simulink model "GuytonModel1986All_R2015a"  (R2015a)
settings: Solver=ode15s  StartTime=0  StopTime=383040  FixedStep=0.03  MaxStep=360  RelTol=1e-3
libraries: simulink x3
(part 1 of 5)
settings Model: Creator=Jirka  LastModifiedBy=User
settings SolverCC: ZeroCrossControl=DisableAll  SolverResetMethod=Robust
settings DataIOCC: SignalLoggingSaveFormat=ModelDataLogs
settings OptimizationCC: ExpressionDepthLimit=2147483647  InitFltsAndDblsToZero=on
settings DebuggingCC: AlgebraicLoopMsg=error  ArtificialAlgebraicLoopMsg=error  SaveWithParameterizedLinksMsg=none  UnderspecifiedInitializationDetection=Classic  MergeDetectMultiDrivingBlocksExec=none  SignalResolutionControl=TryResolveAllWithWarning  SolverPrmCheckMsg=warning  MultiTaskDSMMsg=warning  MultiTaskCondExecSysMsg=none  FcnCallInpInsideContextMsg=EnableAllAsWarning  StateNameClashWarn=warning
settings GRTTargetCC: TargetFcnLib=ansi_tfl_tmw.mat  GeneratePreprocessorConditionals=Use local settings  CombineOutputUpdateFcns=off  GRTInterface=on

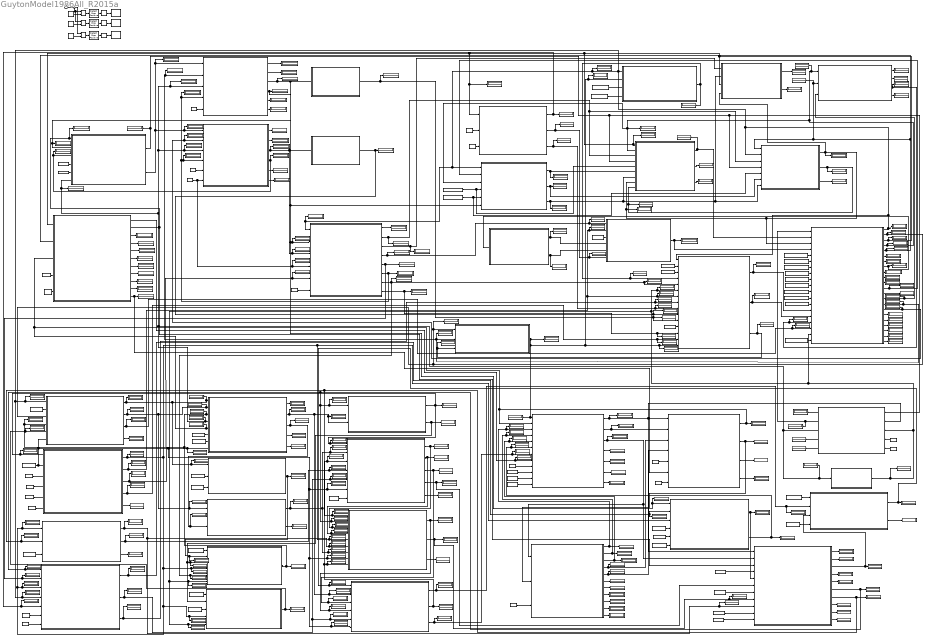
== system GuytonModel1986All_R2015a ==
  note: HSR
  note: HPR
  note: HPL
  2 : Constant
  AARK : Constant  Value=40
  ADH : Constant  Value=0
  AHMRM : Constant  Value=0
  ALCLK : Constant
  ALD : Constant  Value=0
  ANG : Constant  Value=0
  ANUBRM : Constant  Value=0
  ANUVM1 : Constant  Value=0
  ANXM : Constant  Value=0
  ANY : Constant  Value=-0.2
  ATRRFBM : Constant  Value=0
  ATRVFBM : Constant  Value=0
  AUZ : Constant
  Afferent Arteriole : Subsystem
      settings: MinAlgLoopOccurrences=on
      mask Display: disp('AFFERENT ARTERIOLE\n\nINTPUTS:\nAARK - normal resistance in afferent arteriole [torr min/l]\nRNAUG1 - macula densa feedback signal [ratio to normal] \nAUM - sympathetic vasoconstrictor effect on arteries \n[ratio to normal] \nANM - angiotensin multiplier effect on vascular resistance \n[ratio to normal]\nVIM - blood viscosity [ratio to normal blood] \n\n\n OUTPUT:\nAAR - afferent arteriolar resistance [torr l/min]\n')
  Assertion : Assertion  AssertionFailFcn=set_param(bdroot,'SimulationCommand','pause');  StopWhenAssertionFail=off
  Assertion1 : Assertion  AssertionFailFcn=set_param(bdroot,'SimulationCommand','pause');  StopWhenAssertionFail=off
  Assertion2 : Assertion  AssertionFailFcn=set_param(bdroot,'SimulationCommand','pause');  StopWhenAssertionFail=off
  Autonomic Contorl of the Circulation : Subsystem
      mask Display: disp('AUTONOMIC CONTROL OF THE CIRCULATION\n\nINTPUTS:\nPA - systemic arterial pressure torr\nPOT - non-muscle cell PO2 [torr]\nPMO - muscle cells PO2 [torr] \nEXC - Effect of excercise on the metabolic usage of oxygen \nby the muscles [ratio to resting state]\nANUBR - direct effect of angiotensin on vasomotor center \n["virtual" torr]\nAUZ - overall sensitivity of autonomic control [ratio to normal]\n\nOUTPUTs:\nAU - overall activity af autonomic system\n[ratio to normal]\nAUH - autonomic multilier effect on the heart output\n[ratio to normal]\nAUR - autonomic multilier effect on heart rate\n[ratio to normal]\nVVR - basic volume of venous tree(maximum volume\n at zero pressure) [l]\nAUP - autonomic multipllier effect on ADH hormone excretion etc. \n[ratio to normal]\nAOM - autonomic multipllier effect on tissue oxygen utilisation \n[ratio to normal]\nAUM - autonomic multipllier effect on arterial resistance \n[ratio to normal]\nAVE - autonomic multipllier effect on venous resistance\n[ratio to normal]\n')
  Blood viscosity : Subsystem
      settings: MinAlgLoopOccurrences=on
      mask Display: disp('BLOOD VISCOSITY\n\nINTPUT:\nHM - hematocrit [%]\n\nOUTPUT:\nVIM - blood viscosity [ratio to normal]')
  CAS : Constant  Value=0.00355
  "CFC " : Constant  Value=0.01167
  CLA : Constant  Value=0.01
  CPA : Constant  Value=0.0048
  CPF : Constant  Value=0.0003
  CPP : Constant  Value=72
  CRA : Constant  Value=0.005
  CV : Constant  Value=0.0825
  Capillary Membrane Fluid Dynamics : Subsystem
      mask Display: disp('CAPILLARY MEMBRANE FLUID DYNAMICS\n\nINTPUTS:\nPC - systemic capillary pressure [torr]\nPGH - hydrostatic pressure in the tissue gel [torr]\nPPC - plasma colloid osmotic pressure [torr] \nPTC - colloid osmotic pressure of the tissue gel [torr]\nVTL - rate of return of fluid from the interstitium to the\nblood through the lymph [l/min]\nTVD - rate of intake of fluid by mounth or otherwise [l/min]\nVUD - loss of fluid into the urine [l/min]\nDFP - loss of fluid from the pulmonary capillaries [l/min]\nVID - rate of transfer of fluid into the cells [l/min]\nCFC - capillary filtration coefficient [l/min/torr]\n(normal value CFC=0.01167)\nVPN - normal value of plasma volume [l]\nVTSN - normal value of interstitital fluid volume [l]/n\nOUTPUTS:\nVP - plasma volume [l]\nVTS - total interstitial fluid volume [l]\nVTCPL - rate of leakage of whole plasma through \n the capillary membrane [l/min]\nCFILTR - rate of filtration from the systemic capillaries [l/min]\nVTC - toral rate of movement of fluid out of systemic capillaries[l/min]\nVPR - plasma volume [ratio to normal]\nVTS - total interstitial fluid volume [ratio to normal]\n')
  Circulatory Dynamics - Flows And Pressures : Subsystem
      settings: MinAlgLoopOccurrences=on
      mask Display: disp('CIRCULATORY DYNAMICS - FLOWS AND PRESSURES\n\nINPUTS:\nVB - blood volume [l]\nQRO - actual right ventricular output [l/min]\nQLO - output of left ventricle [l/min]\nVVS0 - unstressed venous systemic vascular volume [l]\nVAS0 - unstressed volume in systemic arteries [l]\nVRA0 - unstressed right atrial volume [l]\nVPA0 - unstressed volume in pulmonary arteries [l]\nVLA0 - unstressed volume in left atrium and pulmonary veins [l] \nCAS - capacitance of systemic arteries [l/torr] \nCV - capacitance of venous systemic volume [l/torr] \nCRA - capacitance of right atrium [l/torr]\n CPA - capacitance of pulmonary arteries [l/torr]\n CLA - capacitance of left atrium and pulmonary veins [l/torr] \nRSN - vascular resistance in non-muscle \n and non renal tissues [torr min /l]\nRSM - vascular resistance in muscles [torr min /l]\n RPT -pulmonary vascular resistance [torr min /l] \nRR - total renal resistance [torr min /l]\nVIM - blood viscosity (ratio to normal blood)\nFIS - conductance of the fistula [l/min/torr]\n\nOUTPUTS: \nPA - arterial (aortic) pressure [torr]\nPVS - average venous pressure [torr]\nPRA - right atrial pressure [torr]\nPPA - pulmonary arterial pressure [torr]\nPLA - left atrial pressure [torr]\nVAS - volume in systemic arteries [l]\nVVS - systemic venous vascular volume [l]\nVVE - excess blood volume in the veins [l] \nVRA - right atrial volume [l]\nVPA - volume in pulmonary arteries [l]\nVLA - volume in left atrium [l]\nQAO - blood flow in the systemic arterial system [l/min]\nQVO - rate of blood flow from veins into right atrium [l/min]\nQPO - rate of blood flow into pulmonary veins\n and left atrium [l/min]\nBFN - blood flow in non muscle and non renal tissues [l/min]\nBFM - blood flow in muscles [l/min]\nRBF - renal blood flow [l/min]\nFISFLO - blood flow through a fistula [l/min]\nRTP - total systemic peripheral resistance [torr min /l]\nVT0 - total unstressed blood volume [l]	\nVE0 - total excess volume of blood in the vasculature [l]\nMCP - mean circulatory pressure [torr]\n');
  Clock : Clock
  Constant : Constant  Value=20160
  Constant1 : Constant  Value=40320
  Constant137 : Constant  Value=30240
  DIURET : Constant
  DPR : Constant  Value=0
  DR : Constant  Value=0
  "Delivery of Oxygen to the Muscles " : Subsystem
      settings: MinAlgLoopOccurrences=on
      mask Display: disp('MUSCLE O2 DELIVERY\n\nINTPUTS:\nOVA - oxygen content of arterial blood \n[ml O2 STPD/l blood] \nBFN - blood flow in muscles \n [l/min]\nHM - hematocrit [%]\n    AOM - autonomic effect on tissue oxygenation \n [ratio to normal]\nOMM - basic oxygen utilisation in muscles \n[ml O2 STPD/min]\nEXC - Effect of excercise on the metabolic usage \nof oxygen by the muscles [ratio to resting state]\n\nOUTPUTS:\nOVS - muscle venous oxygen saturation [%]\nPVO - muscle venous PO2 [torr]\nPMO - muscle cell PO2 [torr]\nRMO - rate of oxygen delivery to muscles \n[ml O2 STPD/min]\nMMO - rate of oxygen utilisation by muscles\n[ml O2 STPD/min]\nQOM - muscle total cellular oxygen \n[ml O2 STPPD]\n')
  Delivery of Oxygen to the Non-muscleTtissues : Subsystem
      settings: MinAlgLoopOccurrences=on
      mask Display: disp('NON MUSCLE O2 DELIVERY\n\nINTPUTS:\nOVA - oxygen content of arterial blood \n[ml O2 STPD/l blood] \nBFN - blood flow in non-muscle and non-renal tissues \n [l/min]\nHM - hematocrit [%]\n    AOM - autonomic effect on tissue oxygenation \n[ratio to normal]\nO2M - basic oxygen utilisation in non-muscle cells \n[ml O2 STPD/min]\n\nOUTPUTS:\nOSV - non-muscle venous oxygen saturation [%]\nPOV - non muscle venous PO2 [torr]\nPOT - non muscle cell PO2 [torr]\nDOB - rate of oxygen delivery to non-muscle cells \n[ml O2 STPD/min]\nMO2 - rate of oxygen utilisation by non-muscle tissues \n[ml O2 STPD/min]\nQO2 - non-muscle total cellular oxygen \n[ml O2 STPD]\n')
  Detect Rise Positive : simulink/Logic and Bit Operations/Detect Rise Positive  vinit=0  InputProcessing=Inherited  OutDataTypeStr=boolean
  Detect Rise Positive1 : simulink/Logic and Bit Operations/Detect Rise Positive  vinit=0  InputProcessing=Inherited  OutDataTypeStr=boolean
  Detect Rise Positive2 : simulink/Logic and Bit Operations/Detect Rise Positive  vinit=0  InputProcessing=Inherited  OutDataTypeStr=boolean
  Display{,1..266} (267 alike) : Display
  EARK : Constant  Value=43.333
  EFARF : Constant  Value=0
  EXC : Constant
  Effect of stress relaxation on basic venous volume : Subsystem
      settings: MinAlgLoopOccurrences=on
      mask Display: disp('VENOUS STRESS RELAXATION\n\nINTPUTS:\nVVE - excess blood volume in the veins [l] \n\nOUTPUTS:\nVV6 - increased venous vascular volume \ncaused by long time stress realaxation [l]\nVV7 - - increased venous vascular volume \ncaused by short time stress realaxation [l]\n')
  Efferent Arteriole : Subsystem
      settings: MinAlgLoopOccurrences=on
      mask Display: disp('EFFERENT ARTERIOLE\n\nINTPUTS:\nAARK - normal resistance in efferent arteriole [torr min/l\nRNAUG1 - macula densa feedback signal \nto efferent arteriole [ratio to normal] \nEAFRF - sensitivity contoller of macula densa feedback signal\nto efferent arteriole\nANM - angiotensin multiplier effect on vascular resistance \n[ratio to normal]\nVIM - blood viscosity [ratio to normal blood] \n\n\n OUTPUT:\nAAR - afferent arteriolar resistance [torr l/min]\n')
  Extracellular and Intracellular Fluid Electrolytes and Volumes : Subsystem
      settings: MinAlgLoopOccurrences=on
      mask Display: disp('ECF AND ICF ELECTROLYTES AND VOLUMES\n\nINTPUTS:\nVP - plasma volume [l]\nVTS - systemic interstitial fluid volume [l]\nVPF - pulmonary interstitial fluid volume [l]\nNID - normal rate of sodium intake [mmol/min]\nSTH - salt appetite multiplier factor [ratio to normal]\nNOD - rate of excretion of sodium in the urine [mmol/min]\nKID - rate of intake of potassium [mmol/min]\nKOD - rate of excretion of potassium in the urine [mmol/min]\nAMK - aldosterone multiplier factor for the effect of aldosterone \n on the transport of potassium\n through the cell membrane [ratio of normal effect]\nACLK - sensitivity control of the effect of the aldosterone \n on cellular membrane transport\n of potassium [ratio of normal effect]\nVICnorm - normal value of the intracellular fluid volume [l]\n \nOUTPUTS:\nVEC - volume of extracellular fluid [l]\nVIC - volume of intracellular fluid [l]\nVTW - total body water [l]\nVID - rate of fluid transfer between interstitial fluid and cells [l/min]\nNAE - total extracellular sodium content [mmol]\nCNA - extracellular sodium concentration [mmol/l]\nCKE - extracellular potassium concentration [mmol/l]\nKI - total intracellular potassium content [mmol]\nCKI - intracellular potassium concentration [mmol/l]\nKCD - rate of transferof potassium from the interstitial fluid \ninto the intracellular fluid [mmol/min]\n')
  FIS : Constant  Value=0
  GBL : Constant  Value=0
  GLFC : Constant  Value=0.0208
  Glomerulus : Subsystem
      settings: MinAlgLoopOccurrences=on
      mask Display: disp('GLOMERULUS\n\nINTPUTS:\nPAR - renal perfusion pressure[torr]\nRFN - renal blood flow if kidney is not damaged [l/min] \nAAR - resistance in afferent arteriole \n[torr min/ll] \nHM - hematocrit \nPPC - plasma colloid osmotic pressure [torr]\nPXTP - back pressurein proximal tubule [torr]\nGLFC - glomerular filtration coefficient [l/torr/min]\nREK - percent of normal renal function [ratio to normal] \n\n\n OUTPUTS:\nGFR - glomerular filtration rate [l/min]\nGFN - glomerular filtration rate if kidney is not damaged [l/min]\nGLP - glomerular pressure [torr]\nGLPC - average glomerular plasma colloid osmotic pressure [torr]\nPFL - net pressure gradient in glomerulus [torr]\n')
  HSL : Constant
  HSR : Constant
  Heart Rate and Stroke Volume : Subsystem
      settings: MinAlgLoopOccurrences=on
      mask Display: disp('HEART RATE AND STROKE VOLUME\n\nINTPUTS:\nAUR - autonomic stimulation of heart rate \n[ratio to normal] \nHMD - cardiac depresant effect of hypoxia, shock\nand other factors [ratio to normal] \nPRA - right atrial pressure [torr]\nQLO - output of left ventricle [l/min]\n\nOUTPUTS:\nHR - heart rate [beats/min]\nSVO - stroke volume [l]\n')
  Heart hypertrophy or deterioration : Subsystem
      settings: MinAlgLoopOccurrences=on
      mask Display: disp('HEART HYPERTROPHY OR DETERIORATION\n\nINTPUTS:\nPA - systemic arterial pressure [torr]\nQAO - blood flow in the systemic arteriel system [l/min]\nPPA - pulmonary arterial pressure [torr]\nHSR - basic strenght or right ventricle [ratio to normal]\nHSL - basic strenght or left ventricle [ratio to normal]\nPOT - Non muscle cells PO2 [troo]\n\nOUTPUTS:\nHPR - hypertrophy effect of right heart [ratio to normal]\nHPL - hypertrophy effect of left heart [ratio to normal]\nHMD - cardiac depresant effect of hypoxia, shock\n')
  "Interstitial Tissue Fluids, Pressures and Gel Dynamics" : Subsystem
      mask Display: disp('INTERSTITIAL TISSUE FLUIDS, PRESSURES AND PROTEIN DYNAMICS\n\nINTPUTS:\nVTS - total interstitial fluid volume [l]\nDPC -rate of influx protein into the interstitial fluid from plasma [g/min]\nTSP0 - initial value of total interstitial tissue proteins [g]\n\nOUTPUTs:\nPGH - hydrostatic pressure in tissue gel [torr]\nPTC - total colloid osmotic pressure of the tissue gel]\nVTL - lymph flow rate [l/min]\nDPL - rate of return of protein to the circulatin by way of the lymph [g/min]\nCPI - concentration pf protein in the interstitium [g/l]\nPTT - total interstitial tissue pressure [torr]\nPIF - pressurte in the free interstitial fluid [torr]\nPTS - solid tissue pressure [torr]\nVIF - free interstitial fluid volume[l]\nVG - tissue gel volume[l]\nTSP - total interstitial tissue proteins [g]\n')
  KID : Constant  Value=0.06
  LPPR : Constant  Value=0.03
  Left Heart Pumping : Subsystem
      settings: MinAlgLoopOccurrences=on
      mask Display: disp('LEFT HEART PUMPING\n\nINTPUTS:\nPLA - left atrial pressure [torr]\nPA - systemic arterial pressure [torr]\nAUH - autonomic stimulation of heart [ratio to normal] \nOSA - oxygen hemoglobin saturation \nHSL - basic strenght or left ventricle (ratio to normal)\nHPL - hypertrophy effect of left heart [ratio to normal]\nHMD - cardiac depressant effect of hypoxia, shock \n and other factors [ratio to normal]\n\nOUTPUTS:\nQLO - actual left ventricular output [l/min]\nQLN - normalised lwft ventricular output [l/min]\nLVM - depressing effect on left ventricle of pulmonary \n arterial pressure [ratio to normal]\n')
  Logical Operator : Logic  Operator=NOT  AllPortsSameDT=off  OutDataTypeStr=boolean
  Logical Operator1 : Logic  Operator=NOT  AllPortsSameDT=off  OutDataTypeStr=boolean
  Logical Operator2 : Logic  Operator=NOT  AllPortsSameDT=off  OutDataTypeStr=boolean
  MYOGTAU : Constant  Value=240
  MYOGTAU1 : Constant  Value=240
  Macula densa : Subsystem
      settings: MinAlgLoopOccurrences=on
      mask Display: disp('MACULA DENSA\n\nINTPUTS:\nCNA - Extracellular sodium concentration [mmol/l]\nGFN - glomerular filtration rate if kidney \nis not damaged [l/min]\n\n\n OUTPUTS:\nRNAUG1 - macula densa feedback signal \n[ratio to normal effect]\nNAPT1 - delivery of sodium to the macula densa area \n[ratio to normal value]\n')
  "Muscle Local Blood Flow Control " : Subsystem
      settings: MinAlgLoopOccurrences=on
      mask Display: disp('MUSCLE LOCAL BLOOD FLOW CONTROL\n\nINTPUT:\nPMO - muscle cells PO2 [torr] \n\nOUTPUT:\nAMM - vasoconstrictor effect of local blood flow\n autoregulationin muscles\n[ratio to normal]\n')
  Myogenic Autoregulation : Subsystem
      settings: MinAlgLoopOccurrences=on
      mask Display: disp('MYOGENIC AUTOREGULATION\n\nINTPUTS:\nPA -  systemic arterial pressure [torr]\nPC - capillary pressure [torr]\nMYOGTAU - time delay factor of myogenic response \n(in normal condition TENSTC= 240 min)\nTENSGN - factor of effectiveness of myogenic response\n \n\n OUTPUT:\nMYOGRS - myogenic autoregulation effect on vascular resistance \n  in muscle and in non-renal tissue [multiplier, ratio to normal]\n')
  Myogenic Autoregulation of Afferent Arteriole : Subsystem
      settings: MinAlgLoopOccurrences=on
      mask Display: disp('MYOGENIC AUTOREGULATION OF AFFERENT ARTERIOLE\n\nINTPUTS:\nPAR - renal perfusion pressure [torr]\nPC - capillary pressure [torr]\nMYOGTAU - time delay factor of myogenic response \n(in normal condition TENSTC= 240 min)\nTENSGN - factor of effectiveness of myogenic response\n \n\n OUTPUT:\nMYOGRSAA - myogenic autoregulation effect on vascular resistance \n  in afferent arteriole [multiplier, ratio to normal effect]\n')
  NID : Constant  Value=0.1875
  "Non-muscle Local Blood Flow Control " : Subsystem
      settings: MinAlgLoopOccurrences=on
      mask Display: disp('NON MUSCLE LOCAL BLOOD FLOW CONTROL\n\nINTPUT:\nPOT - non-muscle cells PO2 [torr] \n\nOUTPUT:\nARM - vasoconstrictor effect of local blood flow\n autoregulationin non-muscle tissues \n[ratio to normal]\n')
  O2M : Constant  Value=164.5
  OMM : Constant  Value=60
  PLURCNORM : Constant  Value=4
  PO2AMB : Constant  Value=150
  PO2DFF : Constant
  PXTP : Constant  Value=8
  Peritubular Capillaries : Subsystem
      settings: MinAlgLoopOccurrences=on
      mask Display: disp('PERITUBULAR CAPILLARIES\n\nINTPUTS:\nRFN - renal blood flow if kidney is not damaged [l/min] \nGLPC - average glomerular plasma colloid osmotic pressure [torr]\n\n\n OUTPUTS:\nRFAB - the multiplier factor for the effect of renal hemodynamics\non reabsorbtion of sodium and potassium\n in the distal tubule collecting duct \n[ratio to normal]\nRCPRS - renal capillary pressure around the tubular systewm [torr]\n')
  Plasma Protein Dynamics : Subsystem
      mask Display: disp('PLASMA PROTEINS DYNAMICS\n\nINTPUTS:\nVP - plasma volume [l]\nVTCLP - rate of leakage of whole plasma through\nthe capillary membrane [l/min]\nDPL - rate of return of protein to the circulation through the lymph [g/min]\nCPI - concentration of protein in the interstitium [g/l] [torr]\nLPPR - rate of production of protein by the liver [g/min]\nPPD - rate of loss of protein through the pulmonary capillary \nmembrane [g/min]\nDPR - rate of loos of protein through the kidney [g/min]\n\nOUTPUTs:\nPPC - plasma colloid osmotic pressure [torr]\nDPC - rate of influx of protein into interstitial fluid from plasma [g/min]\nCPP - plasma protein concentration [g/l]\nDPL - net rate of protein exchange between liver and plasma [g/min]\n')
  Potassium Excretion : Subsystem
      settings: MinAlgLoopOccurrences=on
      mask Display: disp('POTASSIUM EXCRETION\n\nINTPUTS:\nCKE - extracellular potassium concentration [mmol/l]\nCNA - extracellular sodium concentration [mmol/l]\n NADT - the normalized delivery of sodium to the distal tubular system \n[ratio to normal]\nDTNAI - rate of sodium entry into the distal tubular system [mmol/min]\nANM - angiotensin multilier effect to vascular resistance [ratio to normal]\nAMK - effect of aldosterone on potassium secretion [ratio to normal]\nRFAB - the multiplier factor for the effect of renal hemodynamics\non reabsorbtion of sodium and potassium\n in the distal tubule collecting duct \n[ratio to normal]\nREK - percent of normal renal function [ratio to normal] \nVUDN - rate of urinary output if kidney is not damaged [l/min]\n\n\n OUTPUTS:\nKODN - potassium excretion rate if kidney is not damaged [mmol/min]\nKOD - potassium excretion rate [mmol/min]\nCKU - concentration of potassium in urine [mmol/l]\n')
  Pulmonary Fluid Dynamics : Subsystem
      mask Display: disp('PULMONARY FLUID DYNAMICS\n\nINTPUTS:\nPPA - pulmonary arterial pressure [torr]\nPLA - left atrial pressure [torr]\nPPC - plasma colloid osmotic pressure [torr]\nCPF - pulmonary capillary filtration coeffitient [l/min/torr]\n\nOUTPUTs:\nDFP - rate of change of free fluid in the lungs [l/min]\nVPF - volume of free fluid in the pulmonary interstitium [l/min]\nPCP - pulmonary capillary pressure [torr]\nPOS - osmotic pressure in pulmonary interstitial fluid pressure [torr]\nPPI - pulmonary interstitial fluid pressure [torr]\nPFI - rate of fluid filtration out of pulmonary capillary [l/min]\nPLF - pulmonary lymph flow rate [l/min]\nCPN - concentration of protein in pulmonary interstitial fluid [g/l]\nPPN - protein leakage rate through the pulmonary capillary membrane [g/min]\nPPR - total quantity of protein in pulmonary interstitial fluid [g]\nPPD - rate of loss of protein through the pulmonary capillary \nmembrane [g/min]\n')
  Pulmonary O2 Delivery : Subsystem
      mask Display: disp('PULMONARY O2 DELIVERY\n\nINTPUTS:\nVPF - volume of free fluid in the pulmonary interstitium [l/min]\nDOB - non-muscle oxygen usage[ml/min]\nRMO - muscle oxygen usage [ml/min]\nPO2DEF - normalised difussion coecficient for oxygen\nthrough the pulmonary membrane [at norma PO2DEF=1]\nPO2MAB - ambient oxygen pressure [torr]\nHM - hematocrit\n\nOUTPUTs:\nOSA - arterial oxygen saturation\nOVA - arterial blood oxygen content [ml O2/l blood]')
  RAM : Constant  Value=96.3
  RAR : Constant  Value=30.52
  REK : Constant
  RFN : Constant  Value=1.2
  RVSM : Constant
  Red cells production and destruction : Subsystem
      settings: MinAlgLoopOccurrences=on
      mask Display: disp('RED CELLS PRODUCTION AND DESTRUCTION\n\nINTPUTS:\nOSA - arterial oxygen saturation [ratio to full saturation]\nVP - plasma volume [l]\nVIM - blood viscosity [ratio to normal blood]\nRFN - renal blood flow (if kidney is not damaged) [l/min]\nREK - fraction of normal kidney mass [ratio to normal]\n\nOUTPUTS:\nVRC - volume of red blood cells [l]\nVB - volume of blood [l]\nHM - hematocrit [%]\nRC1 - red cells production rate [l/min]\nRC2 - red cells destruction rate [l/min]\n')
  Relational Operator : RelationalOperator  Operator=>  OutDataTypeStr=boolean
  Relational Operator1 : RelationalOperator  Operator=>  OutDataTypeStr=boolean
  Relational Operator2 : RelationalOperator  Operator=>  OutDataTypeStr=boolean
  Renal Perfusion : Subsystem
      settings: MinAlgLoopOccurrences=on
      mask Display: disp('RENAL PERFUSION\n\nINTPUTS:\nPA - systemic arterial pressure[torr]\nGBL - pressure drop in renal artery \ncaused renal arterial constriction [torr] \nPVS - average systemic venous pressure [torr]\nAAR - resistance in afferent arteriole \n[torr min/ll] \nEAR - resistance in efferent arteriole \n[torr min/ll] \nREK - percent of normal renal function [ratio to normal] \n\n\n OUTPUTS:\nPAR - renal perfusion pressure [torr]\nRFN - renal blood flow if kidney is not damaged [l/min]\nRBF - renal blood flow [l/min]\nRR - renal resistance [torr min/l]\n')
  Resistances in the Pulmonary Circulation and Pulmonary Venous Pressure : Subsystem
      mask Display: disp('RESISTANCES IN THE PULMONARY CIRCULATION \nAND PULMONARY VENOUS PRESSURE\n\nINTPUTS:\nPPA - pulmonary arterial pressure [torr]\nPLA - left atrial pressure [torr]\nQPO - rate of blood flow into pulmonary veins and left atrium [l/min] \n\n\n OUTPUTS:\nRPA - pulmonary arterial resistance [torr min/l]\nRPV - pulmonary venous resistance [torr min/l]\nRPT - total pulmonary vascular resistance [torr min/l]\nPVP - pulmonary venous pressure [torr]')
  "Resistances in the Systemic Circulation " : Subsystem
      settings: MinAlgLoopOccurrences=on
      mask Display: disp('RESISTANCES IN THE SYSTEMIC CIRCULATION \n\nINTPUTS:\nPA - systemic arterial pressure [torr]\nRAM - basic vascular resistance of muscles [torr min/l]\nRAR - basic vascular resistance of non-muscle and non-renal \ntissues [torr min/l]\nMYOGRS - myogenic autoregulation effect on vascular resistance\n in muscle and in non-renal tissue (multiplier, ratio to normal)  \nAUM - sympathetic vasoconstrictor effect on arteries \n in muscle and non-renal tissues\n [multiplier factor, ratio to normal]\nVIM - blood viscosity [ratio to normal]\nANU - nonrenal effect of angiotensin [ratio to normal]\nAHM - antidiuretic hormone effect to non renal vascular \n resistance, multiplier (ratio to normal effect)\n ATRRFB - multiplier factor for the effect on muscle and \nnon-renal vacular resistance of feedback from the atrial \nstretch receptors [multiplier, ratio to resting state]\nAMM - muscle vascular constriction caused by local \ntissue control [multiplier, ratio to resting state)\nARM - the degree of vasoconstrictor effect of autoregulation in \nnon-muscle and non-renal tissues [multilier, ratio to normal]\nRVSM - basal systemic venous multiplier causes basal vascular \n stretch in the venous system [ratio to normal]\nAVE - multiplier factor for the effect of the autonomic nervous system\n on venous resistance [ratio to basal effect]\nANUVN multiplier factor for the effect of angiotensin \n on venous resistance [ratio to normal]\nPC - systemic caplillary pressure [torr]\n\n\n OUTPUTS:\nRSN - vascular resistance in non-muscle and non-renal tissues [torr min/l]\nRSM - vascular resistrance in muscles [torr min/l]\nRVS - resistance in small veins [torr min/l]\n')
  Right Heart Pumping : Subsystem
      settings: MinAlgLoopOccurrences=on
      mask Display: disp('RIGHT HEART PUMPING\n\nINTPUTS:\nPRA - right atrial pressure [torr]\nPPA - pulmonary arterial pressure [torr]\nAUH - autonomic stimulation of heart [ratio to normal] \nOSA - oxygen hemoglobin saturation \nHSR - basic strenght or right ventricle [ratio to normal]\nHPR - hypertrophy effect of heart [ratio to normal]\nHMD - cardiac depressant effect of hypoxia. shock \n and other factors [ratio to normal]\nQLO - output of left ventricle [l/min]\nQLN - normalised output of the left heart [l/min]\n\nOUTPUTS:\nQRO - actual right ventricular output [l/min]\nQRN - normalised right ventricular output [l/min]\nRVM - depressing effect on right ventricle of pulmonary \n arterial pressure [ratio to normal]\n')
  STHENABLED : Constant  Value=0
  Sodium Excretion : Subsystem
      settings: MinAlgLoopOccurrences=on
      mask Display: disp('SODIUM EXCRETION\n\nINTPUTS:\nNAPT1 - delivery of sodium to the macula densa area\n[ratio to normal]\nRFAB - the multiplier factor for the effect of renal hemodynamics\non reabsorbtion of sodium and potassium\n in the distal tubule collecting duct \n[ratio to normal]\nVUDN - rate of urinary output if kidney is not damaged [l/min]\nAMNA - aldosterone for control of sodium reabsorbtion\n[ratio to normal effect] \nAHM - antidiuretic hormone  \n[ratio to normal effect] \nREK - percent of normal renal function [ratio to normal] \nDIURET - effect of diuretic on the distal tubule collecting duct\n[ratio to normal - without diuretics]\n\n\n OUTPUTS:\nNADT - the normalized delivery of sodium to the distal tubular system \n[ratio to normal]\nDTNAI - rate of sodium entry into the distal tubular system [mmol/min]\nNODN - sodium excretion rate if kidney is not damaged [mmol/min]\nNOD - sodium excretion rate [mmol/min]\nCNU - concentration of sodium in urine [mmol/l]\n')
  Systemic Capillary Pressure : Subsystem
      settings: MinAlgLoopOccurrences=on
      mask Display: disp('SYSTEMIC CAPILLARY PRESSURE\n\nINTPUTS:\nPVS - average of systemic venous pressure [torr]\nBFN - blood flow in non-renal and non-muscle tissues [l/min] \nRVS - resistancein small veins [torr min/l]\n\n\n OUTPUT:\nPC - systemic caplillary pressure [torr]\n')
  TENSG : Constant
  TENSGN : Constant
  TSP0 : Constant  Value=278.6
  TVDENABLED : Constant
  The control Functions of Aldosterone : Subsystem
      settings: MinAlgLoopOccurrences=on
      mask Display: disp('THE CONTROL FUNCTIONS OF ALDOSTERONE\n\nINTPUTS:\nANM - angiotensin multiplier effect on vascular resistance \n[ratio to normal value]\nCKE - extracelullar fluid potassium concentrastion [mmol/l] \nALD - rate of infusion of aldosterone \n[relative to normal rate of aldosterone secretion]\n \n\n OUTPUTS:\nAMK - effect of aldosterone on potassium secretion [ratio to normal]\nAMNA - aldosterone for control of sodium reabsorbtion\nAMC - aldosterone concentration [ratio to normal]/n')
  The control Functions of Angiotensin : Subsystem
      settings: MinAlgLoopOccurrences=on
      mask Display: disp('THE CONTROL FUNCTIONS OF ANGIOTENSIN\n\nINTPUTS:\nNAPT1 - delivery of sodium to the macula densa area \n[ratio to normal value]\nREK - percent of normal renal function [ratio to normal] \nANXM - controls of degree of hypertrophy of the juxtaglomerulal\n apparatus [0 = no hypertrophy]\n ANG - excess of angiotensin concentration caused by infusion\n [ratio to normal level of angiotensin]\nANUBRM - sensitivity contoller for the effect of angiotensin \nof the baroreceptor system \nANUVM - sensitivity controller for the multiplier factor \nof the systemic veins \n\n\n OUTPUTS:\nANM - angiotensin multilier factor on vascular resistance [ratio to normal]\nANU - angiotensin multilier factor on peripheral \narteriolar resistance [ratio to normal]\nANUBR - angiotensin multilier factor for the effect in controlling \nthe sensitivity of the baroreceptor system[ratio to normal]\nANUVM - angiotensin multilier factor for the constriction \nof systemic veins [ratio to normal]\nANC - angiotensin concentration in blood [ratio to normal]\n')
  The control Functions of Antitiuretic Hormone : Subsystem
      settings: MinAlgLoopOccurrences=on
      mask Display: disp('THE CONTROL FUNCTIONS OF ANTIDIURETIC HORMONE\n\nINTPUTS:\nCNA - Concentration of sodium in extracelullar fluid [mmol/l]\nAUP - autonomic multipllier effect on ADH hormone excretion etc. \n[ratio to normal]\nANM - angiotensin multiplier effect [ratio to normal]\nPA - systemic arterial pressure [torr]\nH7 - effect of right atrial volume receptor reflex on ADH\n secretion [relative additive factor, normal value = 0] \nAHMRM - sensitivity coefficient for the effect of ADH \non systemic arterial resistance.\n\n\n OUTPUTS:\nAHC1 - antidiuretic hormone concentration \nin the circulating body fluids [ratio to normal]\n AHM - antidiuretic hormone multiplier [ratio to normal effect]\nAHMR - effect of antidiuretic on systemic arterial resistance\n [ratio to normal effect]\nANUBRM - sensitivity contoller for the effect of angiotensin \nof the baroreceptor system \nANUVM - sensitivity controller for the multiplier factor \nof the systemic veins \n')
  The volume receptor feedback mechanism : Subsystem
      mask Display: disp('THE VOLUME RECEPTOR FEEDBACK MECHANISM\n\nINPUTS:\nPRA - riight atrial pressure [torr]\nATRVHBM - sensitivity controller of volumereceptor feedback effect \n on change of basic of venous system\n [ATRVFB=AH7*ATRRVBM, no effect = 0] \nATRRFBM - sensitivity controller of volumereceptor feedback effect \n on nonmuscle arterial resistance \n[ATRRFB=AH7*ATRRFBM, no effect = 0] \n\nOUTPUTS:\nAH7 - effect of right atrial volume receptor reflex on ADH\n secretion [relative additive factor, normal value = 0] \nATRVFB - change in basic volume of venous system \n  caused by atrial volume receptor feedback \nATRRFB - multiplier factor for the effect on muscle and \nnon-renal vacular resistance of feedback from the atrial \nstretch receptors [multiplier, ratio to resting state]\n')
  "Thirst, Drinking and Salt Appetite" : Subsystem
      settings: MinAlgLoopOccurrences=on
      mask Display: disp('THIRST,DRINKING AND SALT APPETITE\n\nINTPUTS:\nPOT - non-muscle cell PO2 [torr]\nAHC1 - antidiuretic hormone concentration factor \nin the circulating body fluids [ratio to normal]\n ANM - angiotensin multilier effect to vascular resistance [ratio to normal]\nAMK - effect of aldosterone on potassium secretion [ratio to normal]\nDR - forced input of fluid over and above the natural drinking desire \n(it may be used for intravenous infusion as well)    [l/min]\nSTHENABLED - switching variable:\nif STHENABLED<=0, then STH is not calcultated and STH=1\n    TVDENABLED - switching variable: \nif TVDENABLED <=0 then TVD is not calculated and TVD=DR\n\n\n OUTPUTS:\nSTH - salt appetite multiplier factor [ratio to normal]\nTVD - actual rate of fluid intake [l/min]\n')
  URFORM : Constant  Value=0.24
  Unstressed volume in systemic venous tree : Subsystem
      settings: MinAlgLoopOccurrences=on
      mask Display: disp('UNSTRESSED SYSTEMIC VENOUS VOLUME\n\nINPUTS:\nVVR - normal maximum volume of blood \n  in the venous system at zero pressure [l]\nANU - nonrenal effect of angiotensin [ratio to normal] \nANY - sensitivity of large veins to effect of angiotensin \n[normal value = -0.2 l/unit of angiotensin]\nVV6, VV7 - changes in basic volume of venous system \n  cauused by stress relaxation [l]\nATRVFB - change in basic volume of venous system \n  caused by atrial volume receptor feedback \n\nOUTPUT:\nVVS0 - the maximum volume ov venous system at zero volume\n (so called unstressed venous volume) [l]')
  Urea : Subsystem
      settings: MinAlgLoopOccurrences=on
      mask Display: disp('UREA\n\nINTPUTS:\nURFORM - rate of urea metabolic production [mmol/min]\nUROD -rate of urea excretion[mmol/min]\nVTW - total body water volume [l]\nPLURCNORM - normal value of urea concentration in body fluids [4 mmol/l]\n\nOUTPUTS:\nPLURC - concentration of urea in body fluids [mmol/l]\nPLUR - total body urea content[mmol/l]\n')
  Urea and Water Excretion : Subsystem
      settings: MinAlgLoopOccurrences=on
      mask Display: disp('UREA AND WATER EXCRETION\n\nINTPUTS:\nPLURC - concentration of urea in body fluids [mmol/l]\nGFN - glomerular filtration rate if kidney is not damaged [l/min]\nNADT - the normalized delivery of sodium to the distal tubular system \n[ratio to normal]\nNODN - sodium excretion rate if kidney is not damaged [mmol/min]\nKODN - potassium excretion rate if kidney is not damaged [mmol/min]\nDTNAI - rate of sodium entry into the distal tubular system [mmol/min]\nAHM - antidiuretic hormone [ratio to normal]\nREK - percent of normal renal function [ratio to normal] \n\n\n OUTPUTS:\nUROD - urea excretion rate [mmol/min]\nVUDN - rate of urinary output if kidney id not damaged [l/min]\nVUDN - rate of urinary output [l/min]\n')
  VAS0 : Constant  Value=0.495
  VICnorm : Constant  Value=25
  VID : Constant  Value=0
  VLA0 : Constant  Value=0.4
  VPA0 : Constant  Value=0.30625
  VPN : Constant  Value=3
  VRA0 : Constant  Value=0.1
  VTSN : Constant  Value=11.98
  wires:
  ANY/1 -> Unstressed volume in systemic venous tree/3(ANY)
  Effect of stress relaxation on basic venous volume/1(VV6) -> Unstressed volume in systemic venous tree/4(VV6), Display86/1
  Effect of stress relaxation on basic venous volume/2(VV7) -> Display85/1, Unstressed volume in systemic venous tree/5(VV7)
  Unstressed volume in systemic venous tree/1(VVS0) -> Display8/1, Circulatory Dynamics - Flows And Pressures/4(VVS0)
  VAS0/1 -> Circulatory Dynamics - Flows And Pressures/5(VAS0)
  VRA0/1 -> Circulatory Dynamics - Flows And Pressures/6(VRA0)
  VPA0/1 -> Circulatory Dynamics - Flows And Pressures/7(VPA0)
  VLA0/1 -> Circulatory Dynamics - Flows And Pressures/8(VLA0)
  CAS/1 -> Circulatory Dynamics - Flows And Pressures/9(CAS)
  CV/1 -> Circulatory Dynamics - Flows And Pressures/10(CV)
  CRA/1 -> Circulatory Dynamics - Flows And Pressures/11(CRA)
  CPA/1 -> Circulatory Dynamics - Flows And Pressures/12(CPA)
  CLA/1 -> Circulatory Dynamics - Flows And Pressures/13(CLA)
  "Resistances in the Systemic Circulation "/1(RSN) -> Display34/1, Circulatory Dynamics - Flows And Pressures/14(RSN)
  Circulatory Dynamics - Flows And Pressures/1(PA) -> Left Heart Pumping/2(PA), Heart hypertrophy or deterioration/1(PA), Autonomic Contorl of the Circulation/1(PA), Display54/1, Display249/1, Display183/1, The control Functions of Antitiuretic Hormone/4(PA), Display180/1, Renal Perfusion/1(PA), Myogenic Autoregulation/1(PA), "Resistances in the Systemic Circulation "/1(PA), Display/1  "PA"
  Circulatory Dynamics - Flows And Pressures/2(PVS) -> Display1/1, Renal Perfusion/3(PVS), Systemic Capillary Pressure/1(PVS), Display236/1  "PVS"
  Circulatory Dynamics - Flows And Pressures/3(PRA) -> Display3/1, Heart Rate and Stroke Volume/3(PRA), Right Heart Pumping/1(PRA), Display30/1, Display83/1, The volume receptor feedback mechanism/1(PRA), Pulmonary Fluid Dynamics/1(PPA)
  Circulatory Dynamics - Flows And Pressures/4(PPA) -> Display137/1, Right Heart Pumping/2(PPA), Display31/1, Heart hypertrophy or deterioration/3(PPA), Resistances in the Pulmonary Circulation and Pulmonary Venous Pressure/1(PPA), Display246/1  "PPA"
  Circulatory Dynamics - Flows And Pressures/5(PLA) -> Left Heart Pumping/1(PLA), Resistances in the Pulmonary Circulation and Pulmonary Venous Pressure/2(PLA), Display247/1, Pulmonary Fluid Dynamics/2(PLA), Display4/1
  Circulatory Dynamics - Flows And Pressures/6(VAS) -> Display6/1
  Circulatory Dynamics - Flows And Pressures/14(QPO) -> Display139/1, Resistances in the Pulmonary Circulation and Pulmonary Venous Pressure/3(QPO)
  FIS/1 -> Circulatory Dynamics - Flows And Pressures/19(FIS)
  Left Heart Pumping/2(QLN) -> Display25/1, Right Heart Pumping/9(QLN), Display28/1
  Right Heart Pumping/1(QRO) -> Display22/1, Circulatory Dynamics - Flows And Pressures/2(QRO)
  Right Heart Pumping/2(QRN) -> Display23/1
  Right Heart Pumping/3(RVM) -> Display24/1
  Left Heart Pumping/3(LVM) -> Display26/1
  Left Heart Pumping/1(QLO) -> Display27/1, Right Heart Pumping/8(QLO), Display29/1, Circulatory Dynamics - Flows And Pressures/3(QLO), Heart Rate and Stroke Volume/4(QLO)
  Heart hypertrophy or deterioration/2(HPL) -> Left Heart Pumping/6(HPL), Display57/1
  RAM/1 -> "Resistances in the Systemic Circulation "/2(RAM)
  "Resistances in the Systemic Circulation "/2(RSM) -> Display33/1, Circulatory Dynamics - Flows And Pressures/15(RSM)
  Resistances in the Pulmonary Circulation and Pulmonary Venous Pressure/3(RPT) -> Display11/1, Display250/1, Circulatory Dynamics - Flows And Pressures/16(RPT)
  Resistances in the Pulmonary Circulation and Pulmonary Venous Pressure/2(RPV) -> Display36/1
  Resistances in the Pulmonary Circulation and Pulmonary Venous Pressure/1(RPA) -> Display37/1
  Resistances in the Pulmonary Circulation and Pulmonary Venous Pressure/4(PVP) -> Display38/1
  Myogenic Autoregulation/1(MYOGRS) -> Display39/1, Display239/1, "Resistances in the Systemic Circulation "/4(MYOGRS)
  TENSGN/1 -> Myogenic Autoregulation/4(TENSGN)
  MYOGTAU/1 -> Myogenic Autoregulation/3(MYOGTAU)
  Heart Rate and Stroke Volume/1(HR) -> Display40/1
  Heart Rate and Stroke Volume/2(SVO) -> Display41/1
  Circulatory Dynamics - Flows And Pressures/8(VVE) -> Effect of stress relaxation on basic venous volume/1(VVE), Display138/1
  Circulatory Dynamics - Flows And Pressures/7(VVS) -> Display2/1
  Circulatory Dynamics - Flows And Pressures/9(VRA) -> Display9/1
  Circulatory Dynamics - Flows And Pressures/10(VPA) -> Display21/1
  Circulatory Dynamics - Flows And Pressures/11(VLA) -> Display10/1
  Circulatory Dynamics - Flows And Pressures/12(QAO) -> Heart hypertrophy or deterioration/2(QAO), Display7/1
  Circulatory Dynamics - Flows And Pressures/13(QVO) -> Display12/1
  Circulatory Dynamics - Flows And Pressures/17(RBF) -> Display20/1
  Circulatory Dynamics - Flows And Pressures/18(FISFLO) -> Display16/1
  Circulatory Dynamics - Flows And Pressures/19(RTP) -> Display17/1
  Circulatory Dynamics - Flows And Pressures/20(VT0) -> Display18/1
  Circulatory Dynamics - Flows And Pressures/21(VE0) -> Display19/1
  Circulatory Dynamics - Flows And Pressures/22(MCP) -> Display43/1
  Delivery of Oxygen to the Non-muscleTtissues/3(POT) -> Display51/1, "Non-muscle Local Blood Flow Control "/1(POT), Autonomic Contorl of the Circulation/2(POT), Display184/1, "Thirst, Drinking and Salt Appetite"/1(POT), Display185/1, Heart hypertrophy or deterioration/6(POT)
  EXC/1 -> "Delivery of Oxygen to the Muscles "/6(EXC), Autonomic Contorl of the Circulation/4(EXC), Display55/1
  OMM/1 -> "Delivery of Oxygen to the Muscles "/5(OMM)
  "Delivery of Oxygen to the Muscles "/1(OVS) -> Display47/1
  "Delivery of Oxygen to the Muscles "/2(PVO) -> Display45/1
  "Delivery of Oxygen to the Muscles "/3(PMO) -> Display46/1, "Muscle Local Blood Flow Control "/1(PMO), Autonomic Contorl of the Circulation/3(PMO), Display177/1
  "Delivery of Oxygen to the Muscles "/4(RMO) -> Display48/1, Pulmonary O2 Delivery/3(RMO), Display118/1
  "Delivery of Oxygen to the Muscles "/5(MMO) -> Display49/1
  "Delivery of Oxygen to the Muscles "/6(QOM) -> Display50/1
  Heart hypertrophy or deterioration/3(HMD) -> Right Heart Pumping/7(HMD), Left Heart Pumping/7(HMD), Heart Rate and Stroke Volume/2(HMD), Display58/1  "HMD"
  AUZ/1 -> Autonomic Contorl of the Circulation/6(AUZ)
  Autonomic Contorl of the Circulation/7(AUM) -> Display64/1, Display238/1, "Resistances in the Systemic Circulation "/5(AUM), Display200/1, Afferent Arteriole/5(AUM)
  Autonomic Contorl of the Circulation/1(AU) -> Display60/1
  Autonomic Contorl of the Circulation/5(AUP) -> Display15/1, Display182/1, The control Functions of Antitiuretic Hormone/2(AUP)
  Delivery of Oxygen to the Non-muscleTtissues/2(POV) -> Display69/1
  Delivery of Oxygen to the Non-muscleTtissues/1(OSV) -> Display67/1
  Delivery of Oxygen to the Non-muscleTtissues/4(DOB) -> Display68/1, Pulmonary O2 Delivery/2(DOB), Display117/1
  Delivery of Oxygen to the Non-muscleTtissues/5(MO2) -> Display71/1
  Delivery of Oxygen to the Non-muscleTtissues/6(QO2) -> Display72/1
  O2M/1 -> Delivery of Oxygen to the Non-muscleTtissues/5(O2M)
  Red cells production and destruction/1(VRC) -> Display75/1
  Red cells production and destruction/2(VB) -> Display74/1, Circulatory Dynamics - Flows And Pressures/1(VB)
  Blood viscosity/1(VIM) -> Display79/1, Red cells production and destruction/3(VIM), "Resistances in the Systemic Circulation "/6(VIM), Display241/1, Display203/1, Efferent Arteriole/5(VIM), Display201/1, Afferent Arteriole/6(VIM), Circulatory Dynamics - Flows And Pressures/18(VIM)
  RFN/1 -> Red cells production and destruction/4(RFN)
  2/1 -> Red cells production and destruction/5(REK)
  Red cells production and destruction/4(RC1) -> Display78/1
  Red cells production and destruction/5(RC2) -> Display77/1
  Red cells production and destruction/3(HM) -> Display76/1, Blood viscosity/1(HM), Display52/1, Delivery of Oxygen to the Non-muscleTtissues/3(HM), "Delivery of Oxygen to the Muscles "/3(HM), Display120/1, Pulmonary O2 Delivery/6(HM), Display116/1, Display191/1, Glomerulus/4(HM)  "HM"
  Heart hypertrophy or deterioration/1(HPR) -> Right Heart Pumping/6(HPR), Display56/1
  HSR/1 -> Heart hypertrophy or deterioration/4(HSR), Right Heart Pumping/5(HSR)
  HSL/1 -> Heart hypertrophy or deterioration/5(HSL), Left Heart Pumping/5(HSL)  "HSL"
  Circulatory Dynamics - Flows And Pressures/16(BFM) -> Display141/1, "Delivery of Oxygen to the Muscles "/2(BFM), Display122/1
  Circulatory Dynamics - Flows And Pressures/15(BFN) -> Display140/1, Systemic Capillary Pressure/2(BFN), Delivery of Oxygen to the Non-muscleTtissues/2(BFN), Display53/1, Display253/1  "BFN"
  Autonomic Contorl of the Circulation/3(AUR) -> Display59/1, Heart Rate and Stroke Volume/1(AUR)
  "Non-muscle Local Blood Flow Control "/1(" ARM") -> Display44/1, Display243/1, "Resistances in the Systemic Circulation "/11(ARM)
  "Muscle Local Blood Flow Control "/1(" AMM") -> Display73/1, Display242/1, "Resistances in the Systemic Circulation "/10(AMM)
  Autonomic Contorl of the Circulation/4(VVR) -> Display35/1, Unstressed volume in systemic venous tree/1(VVR), Display237/1
  The volume receptor feedback mechanism/3(ATRRFB) -> Display82/1, "Resistances in the Systemic Circulation "/9(ATRRFB), Display84/1
  ATRVFBM/1 -> The volume receptor feedback mechanism/2(ATRVFBM)
  ATRRFBM/1 -> The volume receptor feedback mechanism/3(ATRRFBM)
  The volume receptor feedback mechanism/2(ATRVFB) -> Display81/1, Unstressed volume in systemic venous tree/6(ATRVFB), Display240/1
  The volume receptor feedback mechanism/1(AH7) -> Display80/1, Display230/1, The control Functions of Antitiuretic Hormone/5(AH7)
  Autonomic Contorl of the Circulation/8(AVE) -> Display61/1, "Resistances in the Systemic Circulation "/13(AVE), Display244/1
  Autonomic Contorl of the Circulation/6(AOM) -> Display14/1, "Delivery of Oxygen to the Muscles "/4(AOM), Display13/1, Delivery of Oxygen to the Non-muscleTtissues/4(AOM), Display119/1
  Autonomic Contorl of the Circulation/2(AUH) -> Right Heart Pumping/3(AUH), Left Heart Pumping/3(AUH), Display42/1
  RAR/1 -> "Resistances in the Systemic Circulation "/3(RAR)
  RVSM/1 -> "Resistances in the Systemic Circulation "/12(RVSM)
  "Resistances in the Systemic Circulation "/3(RVS) -> Display5/1, Systemic Capillary Pressure/3(RVS), Display254/1
  Capillary Membrane Fluid Dynamics/1(VP) -> Plasma Protein Dynamics/1(VP), Extracellular and Intracellular Fluid Electrolytes and Volumes/1(VP), Red cells production and destruction/2(VP), Display105/1
  "CFC "/1 -> Capillary Membrane Fluid Dynamics/10(CFC)
  VID/1 -> Capillary Membrane Fluid Dynamics/9(VID)
  Capillary Membrane Fluid Dynamics/5(VTC) -> Display93/1
  VPN/1 -> Capillary Membrane Fluid Dynamics/11(VPN)
  VTSN/1 -> Capillary Membrane Fluid Dynamics/12(VTSN)
  Capillary Membrane Fluid Dynamics/6(VPREL) -> Display92/1
  Capillary Membrane Fluid Dynamics/7(VTSREL) -> Display89/1
  Plasma Protein Dynamics/2(DPC) -> "Interstitial Tissue Fluids, Pressures and Gel Dynamics"/2(DPC), Display135/1
  Plasma Protein Dynamics/4(DLP) -> Display107/1
  DPR/1 -> Plasma Protein Dynamics/7(DPR)
  TSP0/1 -> "Interstitial Tissue Fluids, Pressures and Gel Dynamics"/3(TSP0)
  "Interstitial Tissue Fluids, Pressures and Gel Dynamics"/1(PGH) -> Display102/1, Capillary Membrane Fluid Dynamics/3(PGH), Display256/1
  Plasma Protein Dynamics/1(PPC) -> Capillary Membrane Fluid Dynamics/2(PPC), Pulmonary Fluid Dynamics/3(PPC), Display192/1, Glomerulus/5(PPC), Display136/1
  "Interstitial Tissue Fluids, Pressures and Gel Dynamics"/2(PTC) -> Display101/1, Capillary Membrane Fluid Dynamics/4(PTC), Display257/1
  "Interstitial Tissue Fluids, Pressures and Gel Dynamics"/3(VTL) -> Display100/1, Capillary Membrane Fluid Dynamics/5(VTL), Display258/1
  LPPR/1 -> Plasma Protein Dynamics/5(LPPR)
  Plasma Protein Dynamics/3(CPP) -> Display108/1
  "Interstitial Tissue Fluids, Pressures and Gel Dynamics"/4(DPL) -> Plasma Protein Dynamics/3(DPL), Display96/1
  "Interstitial Tissue Fluids, Pressures and Gel Dynamics"/5(CPI) -> Plasma Protein Dynamics/4(CPI), Display97/1
  "Interstitial Tissue Fluids, Pressures and Gel Dynamics"/6(PTT) -> Display87/1
  "Interstitial Tissue Fluids, Pressures and Gel Dynamics"/7(PIF) -> Display90/1
  "Interstitial Tissue Fluids, Pressures and Gel Dynamics"/8(PTS) -> Display91/1
  "Interstitial Tissue Fluids, Pressures and Gel Dynamics"/9(VIF) -> Display94/1
  "Interstitial Tissue Fluids, Pressures and Gel Dynamics"/10(VG) -> Display95/1
  "Interstitial Tissue Fluids, Pressures and Gel Dynamics"/11(TSP) -> Display99/1
  Capillary Membrane Fluid Dynamics/2(VTCLP) -> Plasma Protein Dynamics/2(VTCLP), Display104/1
  Capillary Membrane Fluid Dynamics/4(CFILTR) -> Display98/1
  Capillary Membrane Fluid Dynamics/3(VTS) -> "Interstitial Tissue Fluids, Pressures and Gel Dynamics"/1(VTS), Extracellular and Intracellular Fluid Electrolytes and Volumes/2(VTS), Display103/1
  Pulmonary O2 Delivery/2(OVA) -> Display109/1, Delivery of Oxygen to the Non-muscleTtissues/1(OVA), "Delivery of Oxygen to the Muscles "/1(OVA), Display142/1
  Pulmonary O2 Delivery/1(OSA) -> Right Heart Pumping/4(OSA), Left Heart Pumping/4(OSA), Red cells production and destruction/1(OSA), Display110/1  "OSA"
  PO2DFF/1 -> Pulmonary O2 Delivery/4(PO2DEF)
  PO2AMB/1 -> Pulmonary O2 Delivery/5(PO2AMB)
  CPF/1 -> Pulmonary Fluid Dynamics/5(CPF)
  CPP/1 -> Pulmonary Fluid Dynamics/4(CPP)
  Pulmonary Fluid Dynamics/2(VPF) -> Pulmonary O2 Delivery/1(VPF), Display121/1, Extracellular and Intracellular Fluid Electrolytes and Volumes/3(VPF)
  Pulmonary Fluid Dynamics/10(PPR) -> Display63/1
  Pulmonary Fluid Dynamics/1(DFP) -> Capillary Membrane Fluid Dynamics/8(DFP), Display260/1
  NID/1 -> Extracellular and Intracellular Fluid Electrolytes and Volumes/4(NID)  "NID"
  KID/1 -> Extracellular and Intracellular Fluid Electrolytes and Volumes/7(KID)
  ALCLK/1 -> Extracellular and Intracellular Fluid Electrolytes and Volumes/10(ACLK)
  VICnorm/1 -> Extracellular and Intracellular Fluid Electrolytes and Volumes/11(VICNorm)
  Extracellular and Intracellular Fluid Electrolytes and Volumes/1(VEC) -> Display131/1
  Extracellular and Intracellular Fluid Electrolytes and Volumes/2(VIC) -> Display130/1
  Extracellular and Intracellular Fluid Electrolytes and Volumes/3(VTW) -> Display123/1, Urea/3(VTW)
  Extracellular and Intracellular Fluid Electrolytes and Volumes/4(VID) -> Display124/1
  Extracellular and Intracellular Fluid Electrolytes and Volumes/5(NAE) -> Display125/1
  Extracellular and Intracellular Fluid Electrolytes and Volumes/6(CNA) -> Display126/1, Display181/1, The control Functions of Antitiuretic Hormone/1(CNA), Display214/1, Potassium Excretion/2(CNA), Display204/1, Macula densa/1(CNA)
  Extracellular and Intracellular Fluid Electrolytes and Volumes/7(CKE) -> Display127/1, Display179/1, The control Functions of Aldosterone/2(CKE), Display213/1, Potassium Excretion/1(CKE)
  Extracellular and Intracellular Fluid Electrolytes and Volumes/8(KI) -> Display128/1
  Extracellular and Intracellular Fluid Electrolytes and Volumes/9(CKI) -> Display129/1
  Extracellular and Intracellular Fluid Electrolytes and Volumes/10(KCD) -> Display132/1
  Systemic Capillary Pressure/1(PC) -> Display245/1, "Resistances in the Systemic Circulation "/15(PC), Myogenic Autoregulation/2(PC), Display248/1, Capillary Membrane Fluid Dynamics/1(PC), Display255/1, Display32/1
  Urea/1(PLURC) -> Display133/1, Display223/1, Urea and Water Excretion/1(PLURC)
  Urea/2(PLUR) -> Display134/1
  URFORM/1 -> Urea/1(URFORM)
  PLURCNORM/1 -> Urea/4(PLURCNORM)
  "Thirst, Drinking and Salt Appetite"/1(STH) -> Extracellular and Intracellular Fluid Electrolytes and Volumes/5(STH), Display106/1
  "Thirst, Drinking and Salt Appetite"/2(TVD) -> Display88/1, Capillary Membrane Fluid Dynamics/6(TVD), Display259/1
  DR/1 -> "Thirst, Drinking and Salt Appetite"/4(DR)
  STHENABLED/1 -> "Thirst, Drinking and Salt Appetite"/5(STHENABLED)
  TVDENABLED/1 -> "Thirst, Drinking and Salt Appetite"/6(TVDENABLED)
  Pulmonary Fluid Dynamics/11(PPD) -> Plasma Protein Dynamics/6(PPD), Display62/1
  Pulmonary Fluid Dynamics/3(PCP) -> Display115/1
  Pulmonary Fluid Dynamics/4(POS) -> Display114/1
  Pulmonary Fluid Dynamics/5(PPI) -> Display113/1
  Pulmonary Fluid Dynamics/6(PFI) -> Display112/1
  Pulmonary Fluid Dynamics/7(PLF) -> Display111/1
  Pulmonary Fluid Dynamics/8(CPN) -> Display66/1
  Pulmonary Fluid Dynamics/9(PPN) -> Display65/1
  GBL/1 -> Renal Perfusion/2(GBL)
  Afferent Arteriole/1(AAR) -> Display232/1, Renal Perfusion/4(AAR), Display189/1, Glomerulus/3(AAR), Display187/1
  AARK/1 -> Afferent Arteriole/1(AARK)
  Macula densa/2(RNAUG1) -> Display197/1, Afferent Arteriole/3(RNAUG1), Efferent Arteriole/2(RNAUG1), Display149/1
  Efferent Arteriole/1(EAR) -> Display198/1, Display233/1, Renal Perfusion/5(EAR)
  EARK/1 -> Efferent Arteriole/1(EARK)
  EFARF/1 -> Efferent Arteriole/3(EFARF)
  Myogenic Autoregulation of Afferent Arteriole/1(MYOGRSAA) -> Display196/1, Afferent Arteriole/2(MYOGRSAA), Display220/1
  MYOGTAU1/1 -> Myogenic Autoregulation of Afferent Arteriole/2(MYOGTAU)
  TENSG/1 -> Myogenic Autoregulation of Afferent Arteriole/3(TENSGN)
  PXTP/1 -> Glomerulus/6(PXTP)
  GLFC/1 -> Glomerulus/7(GLFC)
  Glomerulus/1(GFR) -> Display144/1
  Glomerulus/2(GFN) -> Display224/1, Urea and Water Excretion/2(GFN), Macula densa/2(GFN), Display205/1, Display209/1
  Glomerulus/3(GLP) -> Display231/1, Peritubular Capillaries/2(GLPC), Display195/1
  Glomerulus/4(GLPC) -> Display145/1
  Glomerulus/5(PFL) -> Display146/1
  Macula densa/1(NAPT1) -> Display207/1, Sodium Excretion/1(NAPT1), Display148/1, The control Functions of Angiotensin/1(NAPT1), Display262/1
  DIURET/1 -> Sodium Excretion/7(DIURET)
  Sodium Excretion/1(NADT) -> Display215/1, Potassium Excretion/3(NADT), Display152/1
  Sodium Excretion/2(DTNAI) -> Display216/1, Potassium Excretion/4(DTNAI), Display153/1
  Sodium Excretion/3(NODN) -> Display225/1, Urea and Water Excretion/3(NODN), Display151/1
  Sodium Excretion/4(NOD) -> Display150/1, Extracellular and Intracellular Fluid Electrolytes and Volumes/6(NOD)  "NOD"
  Sodium Excretion/5(CNU) -> Display156/1
  Potassium Excretion/1(KODN) -> Display226/1, Urea and Water Excretion/4(KODN), Display147/1
  Potassium Excretion/2(KOD) -> Display155/1, Extracellular and Intracellular Fluid Electrolytes and Volumes/8(KOD), Display261/1
  Potassium Excretion/3(CKU) -> Display157/1
  Urea and Water Excretion/1(UROD) -> Display158/1, Urea/2(UROD), Display252/1
  Urea and Water Excretion/2(VUDN) -> Display222/1, Potassium Excretion/9(VUDN), Display208/1, Sodium Excretion/3(VUDN), Display159/1
  Urea and Water Excretion/3(VUD) -> Display160/1, Capillary Membrane Fluid Dynamics/7(VUD), Display264/1
  Peritubular Capillaries/1(RFAB) -> Display219/1, Potassium Excretion/7(RFAB), Display206/1, Sodium Excretion/2(RFAB), Display265/1
  Renal Perfusion/1(PAR) -> Display154/1, Display190/1, Glomerulus/1(PAR), Myogenic Autoregulation of Afferent Arteriole/1(PAR), Display193/1
  Renal Perfusion/2(RFN) -> Display188/1, Glomerulus/2(RFN), Peritubular Capillaries/1(RFN), Display194/1, Display143/1
  Peritubular Capillaries/2(RCPRS) -> Display163/1
  REK/1 -> The control Functions of Angiotensin/2(REK), Renal Perfusion/6(REK), Display229/1, Glomerulus/8(REK), Display212/1, Sodium Excretion/6(REK), Display228/1, Urea and Water Excretion/6(REK), Display221/1, Potassium Excretion/8(REK)  "REK"
  Renal Perfusion/4(RBF) -> Display165/1
  Renal Perfusion/3(RR) -> Display164/1, Display266/1, Circulatory Dynamics - Flows And Pressures/17(RR)  "RR"
  The control Functions of Angiotensin/1(ANM) -> Display217/1, Potassium Excretion/5(ANM), "Thirst, Drinking and Salt Appetite"/3(ANM), Display199/1, Afferent Arteriole/4(ANM), Display235/1, The control Functions of Antitiuretic Hormone/3(ANM), Display234/1, The control Functions of Aldosterone/1(ANM), Display202/1, Efferent Arteriole/4(ANM), Display168/1  "ANM"
  ANXM/1 -> The control Functions of Angiotensin/3(ANXM)
  ANG/1 -> The control Functions of Angiotensin/4(ANG)
  ANUVM1/1 -> The control Functions of Angiotensin/6(ANUVM)
  ANUBRM/1 -> The control Functions of Angiotensin/5(ANUBRM)
  The control Functions of Angiotensin/2(ANU) -> Display167/1, Unstressed volume in systemic venous tree/2(ANU), Display171/1, "Resistances in the Systemic Circulation "/7(ANU), Display178/1  "ANU"
  The control Functions of Angiotensin/3(ANUBR) -> Display176/1, Autonomic Contorl of the Circulation/5(ANUBR), Display70/1
  The control Functions of Angiotensin/4(ANUVN) -> Display166/1, "Resistances in the Systemic Circulation "/14(ANUVN), Display251/1
  The control Functions of Angiotensin/5(ANC) -> Display169/1  "ANC"
  The control Functions of Aldosterone/1(AMK) -> Display170/1, Display218/1, Potassium Excretion/6(AMK), Extracellular and Intracellular Fluid Electrolytes and Volumes/9(AMK), Display263/1
  The control Functions of Aldosterone/2(AMNA) -> Display210/1, Sodium Excretion/4(AMNA), Display161/1
  ALD/1 -> The control Functions of Aldosterone/3(ALD)
  The control Functions of Aldosterone/3(AMC) -> Display162/1
  ADH/1 -> The control Functions of Antitiuretic Hormone/6(ADH)
  The control Functions of Antitiuretic Hormone/1(AHC1) -> Display173/1, "Thirst, Drinking and Salt Appetite"/2(AHC1), Display174/1  "AHC1"
  The control Functions of Antitiuretic Hormone/2(AHM) -> Display227/1, Urea and Water Excretion/5(AHM), Sodium Excretion/5(AHM), Display211/1, Display172/1
  The control Functions of Antitiuretic Hormone/3(AHMR) -> Display186/1, "Resistances in the Systemic Circulation "/8(AHMR), Display175/1  "AHRM"
  AHMRM/1 -> The control Functions of Antitiuretic Hormone/7(AHMRM)
  Constant/1 -> Relational Operator/2
  Constant137/1 -> Relational Operator1/2
  Relational Operator/1 -> Detect Rise Positive/1
  Detect Rise Positive/1 -> Logical Operator/1
  Logical Operator/1 -> Assertion/1
  Detect Rise Positive1/1 -> Logical Operator1/1
  Logical Operator1/1 -> Assertion1/1
  Relational Operator1/1 -> Detect Rise Positive1/1
  Constant1/1 -> Relational Operator2/2
  Clock/1 -> Relational Operator2/1, Relational Operator1/1, Relational Operator/1
  Relational Operator2/1 -> Detect Rise Positive2/1
  Detect Rise Positive2/1 -> Logical Operator2/1
  Logical Operator2/1 -> Assertion2/1
